simulink model "S_GITHUB"  (R2017a)
settings: Solver=VariableStepAuto  StartTime=0.0  StopTime=20  FixedStep=1e-6  MaxStep=1e-4
values from neighbouring files (symbols this model uses):
  Cinv = 470e-6    (= 0.00047)    [M_GITHUB.m]
  Co = 470e-6    (= 0.00047)    [M_GITHUB.m]
  Den = 1.225    [M_GITHUB.m]
  Dg = 0.390    (= 0.39)    [M_GITHUB.m]
  Dmax = 1    [M_GITHUB.m]
  Jg = 5*0.1    (= 0.5)    [M_GITHUB.m]
  Jm = 5*0.1    (= 0.5)    [M_GITHUB.m]
  KI = 0.0195296    [M_GITHUB.m]
  Ki1 = 1/io_nom    (= 0.0444444444444)    [M_GITHUB.m]
  KP = 1.0672352    [M_GITHUB.m]
  L = 80e-3    (= 0.08)    [M_GITHUB.m]
  Rr = 2.9343    [M_GITHUB.m]
  Rs1 = 2.5    [M_GITHUB.m]
  Ts1 = 1/Fs1    (= 0.0002)    [M_GITHUB.m]
undefined symbols (not defined in the file or in its folder): Ion, Lithium, RL
undefined symbols (not defined in the file): Fs1
libraries: powerlib x18, fuzblock x3, simulink x2, electricdrivelib x1, simulink_extras x1
settings Model: ExtModeTrigDuration=10  Creator=dricl  LastModifiedBy=dricl
settings SolverCC: MaxConsecutiveZCs=10000000
settings OptimizationCC: PassReuseOutputArgsAs=Individual arguments  MaxStackSize=2560
settings DebuggingCC: ParameterTunabilityLossMsg=error
settings HardwareCC: ProdBitPerPointer=32  ProdBitPerSizeT=32  ProdBitPerPtrDiffT=32  ProdLargestAtomicInteger=Long  ProdLargestAtomicFloat=Double  ProdWordSize=32  ProdLongLongMode=on  ProdHWDeviceType=ARM Compatible->ARM Cortex
settings SFSimCC: MATLABDynamicMemAlloc=off
settings RTWCC: SystemTargetFile=ert.tlc  HardwareBoard=TI Concerto F28M35x (ARM Cortex-M3)  TLCOptions=-aInlineSetEventsForThisBaseRateFcn=TLC_FALSE -aSuppressMultiTaskScheduler=TLC_FALSE -aRateBasedStepFcn=1  TemplateMakefile=ert_default_tmf  Description=Embedded Coder  GenerateReport=on  Toolchain=Texas Instruments Code Composer Studio v6 (ARM)  IncludeHyperlinkInReport=on  LaunchReport=on  CreateSILPILBlock=PIL  GenerateTraceInfo=on  GenerateTraceReport=on  GenerateTraceReportSl=on  GenerateTraceReportSf=on  GenerateTraceReportEml=on
settings CodeAppCC: ForceParamTrailComments=on  IgnoreCustomStorageClasses=off  OperatorAnnotations=on  SimulinkDataObjDesc=on  SFDataObjDesc=on  MATLABFcnDesc=on  InsertBlockDesc=on  MATLABSourceComments=on

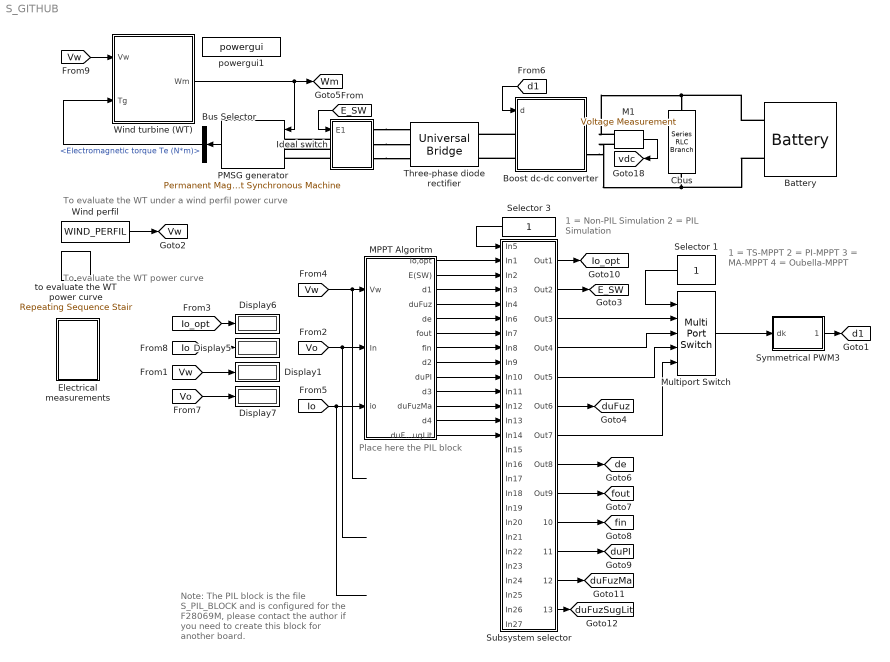
== system S_GITHUB ==
  note: Place here the
      | PIL block
  note: 1 = TS-MPPT
      | 2 = PI-MPPT
      | 3 = MA-MPPT
      | 4 = Oubella-MPPT
  note: 1 = Non-PIL Simulation
      | 2 = PIL Simulation
  note: Note: The PIL block is the file S_PIL_BLOCK and is configured for the F28069M, please contact the author if you need to create this block for another board.
  note: To evaluate the WT under a wind perfil power curve
  note: To evaluate the WT power curve
  Battery : electricdrivelib/Extra Sources/Battery  BatType=Lithium-Ion  ShowTempParam=off  ThermalPreset=no  ShowAgeParam=off  NomV=500  NomQ=5.4  SOC=20  Batt_Tr=30  PresetModel=on  MaxQ=5.4  MinV=375  FullV=581.9936  Dis_rate=2.3478  R=0.92593  Normal_OP=4.8835  expZone="[540.1929     0.2653043]"  current=[6.5 13 32.5]  Units=Time  Tci=20  NomT=20  T2=-30  MaxQ2=4.8  FullV2=7.1  Normal_OP2=5.655  expZone2="[6.58           1]"  Rca=0.6  ti=2000  Dp=0  Neq0=0  Tsim=1e6  Ta1=25  Qeol=5.4*0.9  Reol=0.013333*1.2  Char_age=[2.3478, 3]  Dis_age=[2.3478, 10]  N1=1500  N2=10500  N3=1000  N4=1400  Ta2=45  N5=950
  Boost dc-dc converter : Subsystem
  Bus Selector : BusSelector  OutputSignals=Electromagnetic torque Te (N*m)
  Cbus : powerlib/Elements/Series RLC Branch  LConnTagsString=__new0  RConnTagsString=__new0  BranchType=RC  Resistance=0.01  Inductance=1e-3  SetiL0=off  InitialCurrent=0  Capacitance=Cinv  Setx0=on  InitialVoltage=0  Measurements=None
  Display{1,5..7} (4 alike) : Display
  Electrical measurements : Subsystem
  Ideal switch : Subsystem
  M1 : powerlib/Measurements/Voltage Measurement  PhasorSimulation=off  OutputType=Complex  PSBequivalent=0
  MPPT Algoritm : Subsystem
  Multiport Switch : MultiPortSwitch  Inputs=4
  PMSG generator : powerlib/Machines/Permanent Magnet Synchronous Machine  NbPhases=3  FluxDistribution=Sinusoidal  RotorType=Round  MechanicalLoad=Speed w  PresetModel=No  ShowDetailedParameters=on  MeasurementBus=off  Resistance=Rs1  Inductance=8.5e-3  dqInductances=[0.0007552 0.0008348]  La=La  MachineConstant=Flux linkage established by magnets (V.s)  Flux=Ym  VoltageCst=2176.5592  TorqueCst=18  Flat=120  Mechanical=[0.011 0.001417 4 0]  PolePairs=p  InitialConditions=[0,0, 0,0]  InitialConditions5ph=[0 0 0 0 0 0]  TsPowergui=0  TsBlock=-1  RefAngle=90 degrees behind phase A axis (modified Park)
      settings: SourceProductName=Simscape Power Systems
  Selector 1 : Constant
  Selector 3 : Constant
  Subsystem selector : Subsystem
  Symmetrical PWM3 : Subsystem  AncestorBlock=plecslib_extras2/Modulators/Symmetrical PWM  mask(Symmetrical PWM){sampling=Natural (carrier starts with 0), fc=Fs1, offset=0, input_limits=[0 Dmax], output_values=[0 1]}
      mask prompts: fc "Carrier frequency (Hz):"; offset "Carrier offset (p.u.):"; input_limits "Input limits [min max]:"; output_values "Output values [off on]:"
      mask help: PWM generator with a symmetrical triangular carrier. If the input is a vector, the output is also a vector of the same width.
      mask init:
      | if numel(fc)>1 || fc<=0,
      |   error('Carrier frequency must be a positive scalar.');
      | end
      | if numel(offset)>1 || offset<0 || offset>=1,
      |   error('Carrier offset must be a scalar in the range [0; 1/fc[.');
      | end
      | if sampling == 1,
      |   offset = mod(offset+.75, 1);
      | end
      | 
      | si = [.5 mod(offset, .5)]/fc;
      mask Help: eval('plecs(''help'', ''symmetricalpwm.html'')')
      mask TypeOptions sampling: Natural (carrier starts with 0) | Natural (carrier starts with 1) | Regular (double edge) | Regular (single edge)
  Three-phase diode rectifier : powerlib/Power Electronics/Universal Bridge  Arms=3  SnubberResistance=Rs2  SnubberCapacitance=Cs  Device=Diodes  Ron=Ron  Lon=0  ForwardVoltages="[  0  0  ]"  ForwardVoltage=0.7  GTOparameters=[ 10e-6 , 20e-6 ]  IGBTparameters=[ 1e-6 , 2e-6 ]  Measurements=None  Measurements_2=None  converterType=Rectifier
  Wind perfil : FromWorkspace  VariableName=WIND_PERFIL
  Wind turbine (WT) : Subsystem
      mask Display: image('Rotor.jpg');
  powergui1 : powerlib/powergui  Priority=1  SimulationMode=Continuous  SampleTime=1e-6  frequency=60  Iterations=50  frequencyindice=0  Pbase=100e6  ErrMax=1e-4  UnitsV=kV  UnitsW=MW  buscounter=0  FunctionMessages=off  echomessages=off  EnableUseOfTLC=off  CurrentSourceSwitches=off  DisableSnubberDevices=off  DisableRonSwitches=off  DisableVfSwitches=off  DisplayEquations=off  SolverType=Tustin/Backward Euler (TBE)  Interpol=off  ExternalGateDelay=off  methode=off  Ts=100  x0status=blocks  SPID=on  SwTol=0  HookPort=off  RestoreLinks=warning  ResistiveCurrentMeasurement=off  Frange=[0:2:500]  Ylog=off  Xlog=on  ShowGrid=off  save=off  variable=ZData  structure=0  ZoomFFT=off  StartTime=0.0  cycles=1  DisplayStyle=1  fundamental=60  FreqAxis=off  MaxFrequency=1000  frequencyindicesteady=1  RmsSteady=1  display=off
  to evaluate the WT power curve : simulink/Sources/Repeating Sequence Stair  OutValues=[12 12 14 16 16.8 18 18 14 14 2 2 14 14].'  tsamp=1  OutMin=[]  OutMax=[]  OutDataTypeStr=double  OutputDataTypeScalingMode=double  OutDataType=fixdt(0,8)  ConRadixGroup=Best Precision: Vector-wise  OutScaling=2^-12
  tag scope: E_SW=global, Io_opt=global, Vw=global, Wm=global, d1=global, de=global, duFuz=global, duFuzMa=global, duFuzSugLit=global, duPI=global, fin=global, fout=global, vdc=global
  wires:
  Wind turbine (WT)/1(Wm) -> [Wm], PMSG generator/1
  Bus Selector/1 -> Wind turbine (WT)/2(Tg)  "<Electromagnetic torque Te (N*m)>"
  PMSG generator/1 -> Bus Selector/1
  M1/1 -> [vdc]
  [d1] -> Boost dc-dc converter/1(d)
  [Vw] -> Wind turbine (WT)/1(Vw)
  [Vo] -> Display7/1
  [Vw] -> Display1/1
  [E_SW] -> Ideal switch/1(E1)
  [Io_opt] -> Display6/1
  [Io] -> Display5/1
  [Vw] -> MPPT Algoritm/1(Vw)
  [Io] -> MPPT Algoritm/3(io)
  [Vo] -> MPPT Algoritm/2(In)
  Symmetrical PWM3/1(dmppt) -> [d1]
  Multiport Switch/1 -> Symmetrical PWM3/1(dk)
  Selector 1/1 -> Multiport Switch/1
  MPPT Algoritm/1(Io,opt) -> Subsystem selector/2(In1)
  MPPT Algoritm/2(E(SW)) -> Subsystem selector/3(In2)
  MPPT Algoritm/3(d1) -> Subsystem selector/4(In3)
  MPPT Algoritm/4(duFuz) -> Subsystem selector/5(In4)
  Selector 3/1 -> Subsystem selector/1(In5)
  MPPT Algoritm/5(de) -> Subsystem selector/6(In6)
  MPPT Algoritm/6(fout) -> Subsystem selector/7(In7)
  MPPT Algoritm/7(fin) -> Subsystem selector/8(In8)
  MPPT Algoritm/8(d2) -> Subsystem selector/9(In9)
  MPPT Algoritm/9(duPI) -> Subsystem selector/10(In10)
  MPPT Algoritm/10(d3) -> Subsystem selector/11(In11)
  MPPT Algoritm/11(duFuzMa) -> Subsystem selector/12(In12)
  MPPT Algoritm/12(d4) -> Subsystem selector/13(In13)
  MPPT Algoritm/13(duFuzSugLit) -> Subsystem selector/14(In14)
  ? -> Subsystem selector/15(In15)
  ? -> Subsystem selector/16(In16)
  ? -> Subsystem selector/17(In17)
  ? -> Subsystem selector/18(In18)
  ? -> Subsystem selector/19(In19)
  ? -> Subsystem selector/20(In20)
  ? -> Subsystem selector/21(In21)
  ? -> Subsystem selector/22(In22)
  ? -> Subsystem selector/23(In23)
  ? -> Subsystem selector/24(In24)
  ? -> Subsystem selector/25(In25)
  ? -> Subsystem selector/27(In27)
  Subsystem selector/1(Out1) -> [Io_opt]
  Subsystem selector/2(Out2) -> [E_SW]
  Subsystem selector/3(Out3) -> Multiport Switch/2
  Subsystem selector/4(Out4) -> Multiport Switch/3
  Subsystem selector/5(Out5) -> Multiport Switch/4
  Subsystem selector/6(Out6) -> [duFuz]
  Subsystem selector/7(Out7) -> Multiport Switch/5
  Subsystem selector/8(Out8) -> [de]
  Subsystem selector/9(Out9) -> [fout]
  Subsystem selector/10(Out10) -> [fin]
  Subsystem selector/11(Out11) -> [duPI]
  Subsystem selector/12(Out12) -> [duFuzMa]
  Subsystem selector/13(Out13) -> [duFuzSugLit]
  ? -> Subsystem selector/26(In26)
  Wind perfil/1 -> [Vw]
  connections:
  M1/LConn1 -- Boost dc-dc converter/RConn1 -- Battery/LConn1 -- Cbus/LConn1
  M1/LConn2 -- Boost dc-dc converter/RConn2 -- Battery/LConn2 -- Cbus/RConn1
  Boost dc-dc converter/LConn1 -- Three-phase diode rectifier/RConn1
  Boost dc-dc converter/LConn2 -- Three-phase diode rectifier/RConn2
  Ideal switch/LConn2 -- PMSG generator/LConn2
  Ideal switch/LConn3 -- PMSG generator/LConn3
  Ideal switch/LConn1 -- PMSG generator/LConn1
  Ideal switch/RConn1 -- Three-phase diode rectifier/LConn1
  Ideal switch/RConn2 -- Three-phase diode rectifier/LConn2
  Ideal switch/RConn3 -- Three-phase diode rectifier/LConn3

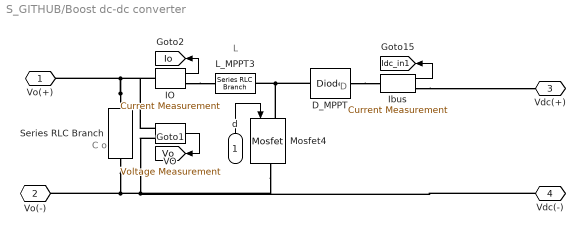
== system S_GITHUB/Boost dc-dc converter ==
  note: C o
  note: L
  note: D
  d : Inport
  D_MPPT : powerlib/Power Electronics/Diode  Ron=0.001  Lon=0  Vf=0.7  IC=0  UseSnubber=0  Rs=1e5  Cs=inf  Measurements=off
  IO : powerlib/Measurements/Current Measurement  PhasorSimulation=off  OutputType=Complex  PSBequivalent=0
  Ibus : powerlib/Measurements/Current Measurement  PhasorSimulation=off  OutputType=Complex  PSBequivalent=0
  L_MPPT3 : powerlib/Elements/Series RLC Branch  LConnTagsString=__new0  RConnTagsString=__new0  BranchType=L  Resistance=RL  Inductance=L  SetiL0=off  InitialCurrent=0  Capacitance=1e-6  Setx0=off  InitialVoltage=0  Measurements=None
  Mosfet4 : powerlib/Power Electronics/Mosfet  Ron=0.001  Lon=0  Rd=0.001  Vfd=0.7  IC=0  Rs=1e5  Cs=inf  Measurements=off
  Series RLC Branch : powerlib/Elements/Series RLC Branch  LConnTagsString=__new0  RConnTagsString=__new0  BranchType=RC  Resistance=0.01  Inductance=1e-3  SetiL0=off  InitialCurrent=0  Capacitance=Co  Setx0=on  InitialVoltage=0  Measurements=None
  VO : powerlib/Measurements/Voltage Measurement  PhasorSimulation=off  OutputType=Complex  PSBequivalent=0
  Vo(+) : PMIOPort  Port=1  Side=Left
  Vo(-) : PMIOPort  Port=2  Side=Left
  Vdc(+) : PMIOPort  Port=3  Side=Right
  Vdc(-) : PMIOPort  Port=4  Side=Right
  tag scope: Idc_in1=global, Io=global, Vo=global
  wires:
  IO/1 -> [Io]
  VO/1 -> [Vo]
  d/1 -> Mosfet4/1
  Ibus/1 -> [Idc_in1]
  connections:
  Ibus/RConn1 -- Vdc(+)/RConn1
  Series RLC Branch/LConn1 -- Vo(+)/RConn1 -- IO/LConn1 -- VO/LConn1
  Series RLC Branch/RConn1 -- Vdc(-)/RConn1 -- Mosfet4/RConn1 -- VO/LConn2 -- Vo(-)/RConn1
  IO/RConn1 -- L_MPPT3/LConn1
  D_MPPT/RConn1 -- Ibus/LConn1
  Mosfet4/LConn1 -- D_MPPT/LConn1 -- L_MPPT3/RConn1

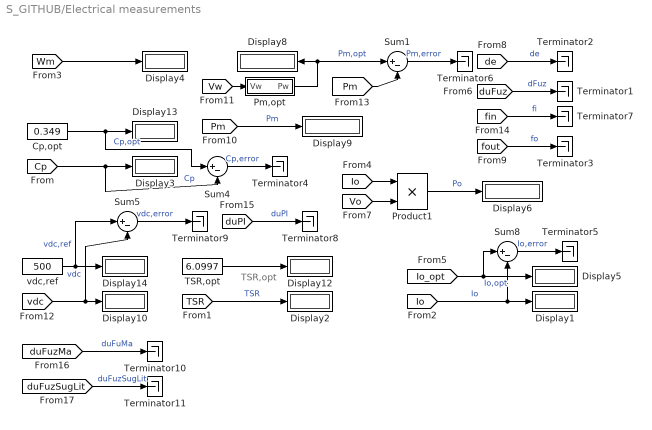
== system S_GITHUB/Electrical measurements ==
  note: TSR,opt
  Cp,opt : Constant  Value=0.349
  Display{1..6,8..10,12..14} (12 alike) : Display
  Pm,opt : MATLAB Function  TreatAsAtomicUnit=on
  Product1 : Product
  Sum{1,4..5,8} (4 alike) : Sum  Inputs=|+-
  TSR,opt : Constant  Value=6.0997
  Terminator{1..11} (11 alike) : Terminator
  vdc,ref : Constant  Value=500
  wires:
  Sum5/1 -> Terminator9/1  "vdc,error"
  vdc,ref/1 -> Sum5/1, Display14/1  "vdc,ref"
  TSR,opt/1 -> Display12/1
  Cp,opt/1 -> Sum4/1, Display13/1  "Cp,opt"
  Sum4/1 -> Terminator4/1  "Cp,error"
  [Pm] -> Sum1/2
  Sum1/1 -> Terminator6/1  "Pm,error"
  [Wm] -> Display4/1
  [TSR] -> Display2/1  "TSR"
  [Cp] -> Sum4/2, Display3/1  "Cp"
  Pm,opt/1(Pw) -> Display8/1, Sum1/1  "Pm,opt"
  [Vw] -> Pm,opt/1(Vw)
  [Pm] -> Display9/1  "Pm"
  [vdc] -> Sum5/2, Display10/1  "vdc"
  [Io_opt] -> Sum8/1, Display5/1  "Io,opt"
  Sum8/1 -> Terminator5/1  "Io,error"
  [Io] -> Sum8/2, Display1/1  "Io"
  [Io] -> Product1/1
  [Vo] -> Product1/2
  Product1/1 -> Display6/1  "Po"
  [duFuz] -> Terminator1/1  "dFuz"
  [de] -> Terminator2/1  "de"
  [fout] -> Terminator3/1  "fo"
  [fin] -> Terminator7/1  "fi"
  [duPI] -> Terminator8/1  "duPI"
  [duFuzMa] -> Terminator10/1  "duFuMa"
  [duFuzSugLit] -> Terminator11/1  "duFuzSugLit"

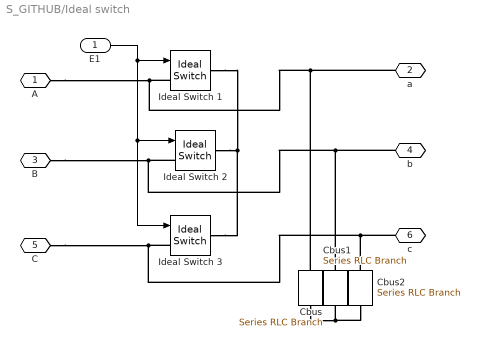
== system S_GITHUB/Ideal switch ==
  E1 : Inport
  Cbus : powerlib/Elements/Series RLC Branch  LConnTagsString=__new0  RConnTagsString=__new0  BranchType=R  Resistance=100000  Inductance=1e-3  SetiL0=off  InitialCurrent=0  Capacitance=Cinv  Setx0=on  InitialVoltage=0  Measurements=None
  Cbus1 : powerlib/Elements/Series RLC Branch  LConnTagsString=__new0  RConnTagsString=__new0  BranchType=R  Resistance=100000  Inductance=1e-3  SetiL0=off  InitialCurrent=0  Capacitance=Cinv  Setx0=on  InitialVoltage=0  Measurements=None
  Cbus2 : powerlib/Elements/Series RLC Branch  LConnTagsString=__new0  RConnTagsString=__new0  BranchType=R  Resistance=100000  Inductance=1e-3  SetiL0=off  InitialCurrent=0  Capacitance=Cinv  Setx0=on  InitialVoltage=0  Measurements=None
  Ideal Switch 1 : powerlib/Power Electronics/Ideal Switch  Ron=0.001  Lon=1e-9  IC=1  Rs=1e6  Cs=100e-9  Measurements=off
      settings: AttributesFormatString=\n
  Ideal Switch 2 : powerlib/Power Electronics/Ideal Switch  Ron=0.001  Lon=1e-9  IC=1  Rs=inf  Cs=0  Measurements=off
      settings: AttributesFormatString=\n
  Ideal Switch 3 : powerlib/Power Electronics/Ideal Switch  Ron=0.001  Lon=1e-9  IC=1  Rs=inf  Cs=0  Measurements=off
      settings: AttributesFormatString=\n
  A : PMIOPort  Port=1  Side=Left
  a : PMIOPort  Port=2  Side=Right
  B : PMIOPort  Port=3  Side=Left
  b : PMIOPort  Port=4  Side=Right
  C : PMIOPort  Port=5  Side=Left
  c : PMIOPort  Port=6  Side=Right
  wires:
  E1/1 -> Ideal Switch 3/1, Ideal Switch 2/1, Ideal Switch 1/1
  connections:
  C/RConn1 -- Ideal Switch 3/LConn1 -- Cbus2/LConn1 -- c/RConn1
  B/RConn1 -- Ideal Switch 2/LConn1 -- Cbus1/LConn1 -- b/RConn1
  A/RConn1 -- Cbus/LConn1 -- a/RConn1 -- Ideal Switch 1/LConn1
  Ideal Switch 1/RConn1 -- Ideal Switch 3/RConn1 -- Ideal Switch 2/RConn1
  Cbus2/RConn1 -- Cbus/RConn1 -- Cbus1/RConn1

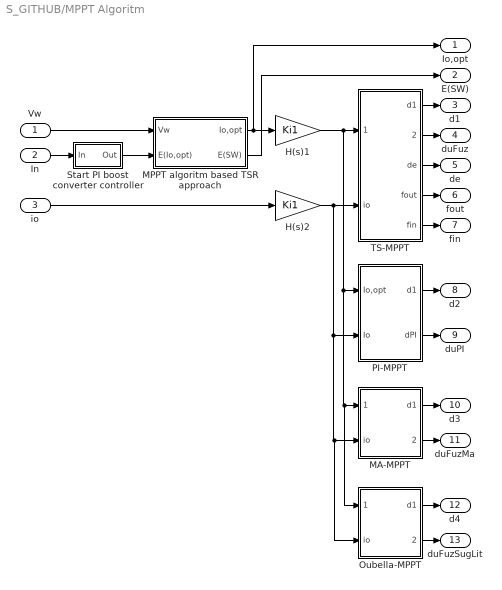
== system S_GITHUB/MPPT Algoritm ==
  Vw : Inport
  In : Inport  Port=2
  io : Inport  Port=3
  H(s)1 : Gain  Gain=Ki1
  H(s)2 : Gain  Gain=Ki1
  MA-MPPT : Subsystem
  "MPPT algoritm based TSR approach " : Subsystem
  Oubella-MPPT : Subsystem
  PI-MPPT : Subsystem
  Start PI boost converter controller : Subsystem
  TS-MPPT : Subsystem
  Io,opt : Outport
  E(SW) : Outport  Port=2
  d1 : Outport  Port=3
  duFuz : Outport  Port=4
  de : Outport  Port=5
  fout : Outport  Port=6
  fin : Outport  Port=7
  d2 : Outport  Port=8
  duPI : Outport  Port=9
  d3 : Outport  Port=10
  duFuzMa : Outport  Port=11
  d4 : Outport  Port=12
  duFuzSugLit : Outport  Port=13
  wires:
  H(s)2/1 -> Oubella-MPPT/2(io), MA-MPPT/2(io), PI-MPPT/2(Io), TS-MPPT/2(io)
  H(s)1/1 -> Oubella-MPPT/1(io,opt), MA-MPPT/1(io,opt), PI-MPPT/1(Io,opt), TS-MPPT/1(io,opt)
  "MPPT algoritm based TSR approach "/1(Io,opt) -> Io,opt/1, H(s)1/1
  io/1 -> H(s)2/1
  "MPPT algoritm based TSR approach "/2(E(SW)) -> E(SW)/1
  Start PI boost converter controller/1(Out) -> "MPPT algoritm based TSR approach "/2(E(Io,opt))
  TS-MPPT/5(fin) -> fin/1
  TS-MPPT/3(de) -> de/1
  TS-MPPT/2(duFuz) -> duFuz/1
  TS-MPPT/4(fout) -> fout/1
  In/1 -> Start PI boost converter controller/1(In)
  Vw/1 -> "MPPT algoritm based TSR approach "/1(Vw)
  TS-MPPT/1(d1) -> d1/1
  PI-MPPT/1(d1) -> d2/1
  PI-MPPT/2(dPI) -> duPI/1
  MA-MPPT/1(d1) -> d3/1
  MA-MPPT/2(duFuzMa) -> duFuzMa/1
  Oubella-MPPT/1(d1) -> d4/1
  Oubella-MPPT/2(duFuzMa) -> duFuzSugLit/1

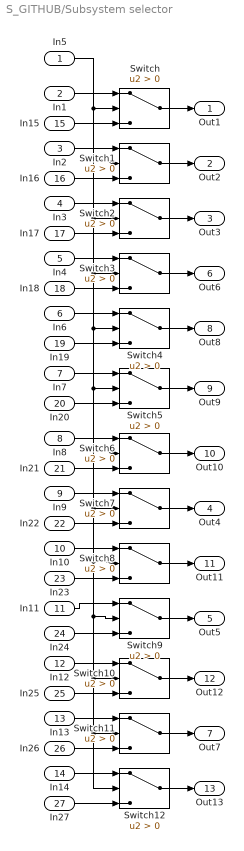
== system S_GITHUB/Subsystem selector ==
  In5 : Inport
  In1 : Inport  Port=2
  In2 : Inport  Port=3
  In3 : Inport  Port=4
  In4 : Inport  Port=5
  In6 : Inport  Port=6
  In7 : Inport  Port=7
  In8 : Inport  Port=8
  In9 : Inport  Port=9
  In10 : Inport  Port=10
  In11 : Inport  Port=11
  In12 : Inport  Port=12
  In13 : Inport  Port=13
  In14 : Inport  Port=14
  In15 : Inport  Port=15
  In16 : Inport  Port=16
  In17 : Inport  Port=17
  In18 : Inport  Port=18
  In19 : Inport  Port=19
  In20 : Inport  Port=20
  In21 : Inport  Port=21
  In22 : Inport  Port=22
  In23 : Inport  Port=23
  In24 : Inport  Port=24
  In25 : Inport  Port=25
  In26 : Inport  Port=26
  In27 : Inport  Port=27
  Switch{,1..12} (13 alike) : Switch  Criteria=u2 > Threshold
  Out1 : Outport
  Out2 : Outport  Port=2
  Out3 : Outport  Port=3
  Out4 : Outport  Port=4
  Out5 : Outport  Port=5
  Out6 : Outport  Port=6
  Out7 : Outport  Port=7
  Out8 : Outport  Port=8
  Out9 : Outport  Port=9
  Out10 : Outport  Port=10
  Out11 : Outport  Port=11
  Out12 : Outport  Port=12
  Out13 : Outport  Port=13
  wires:
  Switch12/1 -> Out13/1
  In26/1 -> Switch11/3
  In13/1 -> Switch11/1
  Switch11/1 -> Out7/1
  In14/1 -> Switch12/1
  Switch9/1 -> Out5/1
  Switch2/1 -> Out3/1
  Switch7/1 -> Out4/1
  In21/1 -> Switch6/3
  In23/1 -> Switch8/3
  Switch/1 -> Out1/1
  Switch4/1 -> Out8/1
  Switch1/1 -> Out2/1
  In11/1 -> Switch9/1
  Switch6/1 -> Out10/1
  Switch8/1 -> Out11/1
  Switch5/1 -> Out9/1
  Switch3/1 -> Out6/1
  In20/1 -> Switch5/3
  In25/1 -> Switch10/3
  In5/1 -> Switch/2, Switch1/2, Switch2/2, Switch3/2, Switch4/2, Switch5/2, Switch6/2, Switch7/2, Switch8/2, Switch9/2, Switch10/2, Switch11/2, Switch12/2
  In27/1 -> Switch12/3
  In16/1 -> Switch1/3
  In12/1 -> Switch10/1
  Switch10/1 -> Out12/1
  In24/1 -> Switch9/3
  In15/1 -> Switch/3
  In6/1 -> Switch4/1
  In9/1 -> Switch7/1
  In10/1 -> Switch8/1
  In17/1 -> Switch2/3
  In8/1 -> Switch6/1
  In18/1 -> Switch3/3
  In3/1 -> Switch2/1
  In2/1 -> Switch1/1
  In4/1 -> Switch3/1
  In7/1 -> Switch5/1
  In1/1 -> Switch/1
  In19/1 -> Switch4/3
  In22/1 -> Switch7/3

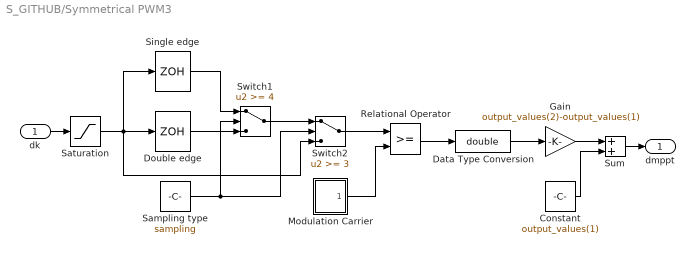
== system S_GITHUB/Symmetrical PWM3 ==
  dk : Inport
  Constant : Constant  Value=output_values(1)
  Data Type Conversion : DataTypeConversion  OutDataTypeStr=double  SaturateOnIntegerOverflow=on  RndMeth=Zero
  Double edge : ZeroOrderHold  SampleTime=si
  Gain : Gain  Gain=output_values(2)-output_values(1)  SaturateOnIntegerOverflow=on  OutDataTypeStr=Inherit: Same as input  ParamDataTypeStr=Inherit: Same as input
  Modulation Carrier : Subsystem  mask(Symmetric Triangle Generator){fc=fc, offset=mod(offset+.5, 1), range=input_limits}
      mask prompts: fc "Carrier frequency (Hz):"; offset "Carrier offset (p.u.):"; range "Signal range [min max]:"
      mask help: Generates a symmetrical triangular signal with output values between 0 and 1. The block forces the Simulink solver to output all tips of the signal. The output can therefore be used as a carrier signal for PWM.
      mask init:
      | if numel(fc)>1 || fc<=0,
      |   error('Carrier frequency must be a positive scalar.');
      | end
      | if numel(offset)>1 || offset<0 || offset>=1,
      |   error('Carrier offset must be a scalar in the interval [0; 1[.');
      | end
      | if numel(range)~=2,
      |   error('Signal range must be a two-element vector.')
      | end
      | if range(1)>=range(2),
      |   error('Signal range must be specified as [min max].')
      | end
      | 
      | carrier_t = [0 offset mod(1/2+offset, 1) 1]/fc;
      | carrier_v0 = 1-2*abs(offset-.5);
      | carrier_v = range(1)+[carrier_v0 0 1 carrier_v0]*diff(range);
      | [carrier_t, idx] = unique(carrier_t);
      | carrier_v = carrier_v(idx);
      | si = [.5 mod(offset, .5)]/fc;
      | 
      | L = length(carrier_t);
      | disp_seq_t = repmat(carrier_t(:),1,3) + ones(L,1)*[0,1,2]/fc;
      | disp_seq_v = repmat(carrier_v(:),1,3);
      mask Display: plot(disp_seq_t, disp_seq_v)
  Relational Operator : RelationalOperator  RndMeth=Nearest  InputSameDT=on
  Sampling type : Constant  Value=sampling
  Saturation : Saturate  UpperLimit=input_limits(2)  LowerLimit=input_limits(1)
  Single edge : ZeroOrderHold  SampleTime=[1 offset]/fc
  Sum : Sum  SaturateOnIntegerOverflow=on  InputSameDT=on  OutDataTypeStr=Inherit: Same as first input
  Switch1 : Switch  Threshold=4  SaturateOnIntegerOverflow=on  InputSameDT=on
  Switch2 : Switch  Threshold=3  SaturateOnIntegerOverflow=on  InputSameDT=on
  dmppt : Outport
  wires:
  Data Type Conversion/1 -> Gain/1
  Constant/1 -> Sum/2
  Gain/1 -> Sum/1
  Sum/1 -> dmppt/1
  Relational Operator/1 -> Data Type Conversion/1
  Switch2/1 -> Relational Operator/1
  Sampling type/1 -> Switch1/2, Switch2/2
  Single edge/1 -> Switch1/1
  Saturation/1 -> Double edge/1, Single edge/1, Switch2/3
  dk/1 -> Saturation/1
  Modulation Carrier/1(Out) -> Relational Operator/2
  Switch1/1 -> Switch2/1
  Double edge/1 -> Switch1/3

== system S_GITHUB/Wind turbine (WT) ==
  Vw : Inport
  Tg : Inport  Port=2
  Theoretical maximum power : MATLAB Function  TreatAsAtomicUnit=on
  WT dynamic model : Subsystem
  WT static model : Subsystem
  Wm : Outport
  tag scope: Cp=global, Pm=global, Pw=global, TSR=global, Tm=global
  wires:
  WT static model/1(Pm) -> [Pm]
  WT static model/3(Cp) -> [Cp]
  WT static model/4(Tm) -> WT dynamic model/1(Tm), [Tm]
  Tg/1 -> WT dynamic model/2(Tg)
  Theoretical maximum power/1(Pw) -> [Pw]
  WT static model/2(TSR) -> [TSR]
  Vw/1 -> Theoretical maximum power/1(Vw), WT static model/1(Vw)
  WT dynamic model/1(Wm) -> WT static model/2(Wm), Wm/1

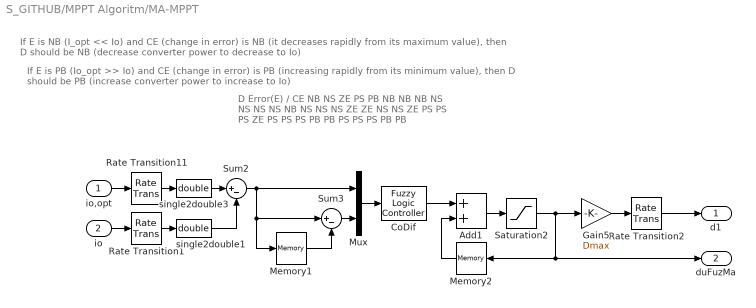
== system S_GITHUB/MPPT Algoritm/MA-MPPT ==
  note: If E is PB (Io_opt >> Io) and CE (change in error) is PB (increasing rapidly from its minimum value), then D should be PB (increase converter power to increase to Io)
  note: If E is NB (I_opt << Io) and CE (change in error) is NB (it decreases rapidly from its maximum value), then D should be NB (decrease converter power to decrease to Io)
  note: D
      | Error(E) / CE NB NS ZE PS PB
      | NB NB NB NS NS NS
      | NS NB NS NS NS ZE
      | ZE NS NS ZE PS PS
      | PS ZE PS PS PS PB
      | PB PS PS PS PB PB
  io,opt : Inport
  io : Inport  Port=2
  Add1 : Sum
  CoDif : fuzblock/Fuzzy Logic  Controller  fis=['MA_MPPT.fis']
  Gain5 : Gain  Gain=Dmax
  Memory1 : Memory  InheritSampleTime=on
  Memory2 : Memory  InheritSampleTime=on
  Mux : Mux  Inputs=2
  Rate Transition1 : RateTransition  Deterministic=off  OutPortSampleTime=Ts6
  Rate Transition11 : RateTransition  Deterministic=off  OutPortSampleTime=Ts6
  Rate Transition2 : RateTransition  Deterministic=off  OutPortSampleTime=Ts6
  Saturation2 : Saturate  UpperLimit=0.98  LowerLimit=0.01
  Sum2 : Sum  Inputs=|+-
  Sum3 : Sum  Inputs=|+-
  single2double1 : DataTypeConversion  OutDataTypeStr=double
  single2double3 : DataTypeConversion  OutDataTypeStr=double
  d1 : Outport
  duFuzMa : Outport  Port=2
  wires:
  Rate Transition2/1 -> d1/1
  Rate Transition11/1 -> single2double3/1
  Sum2/1 -> Sum3/1, Memory1/1, Mux/1
  Memory2/1 -> Add1/2
  single2double3/1 -> Sum2/1
  Mux/1 -> CoDif/1
  Sum3/1 -> Mux/2
  single2double1/1 -> Sum2/2
  Memory1/1 -> Sum3/2
  Rate Transition1/1 -> single2double1/1
  io,opt/1 -> Rate Transition11/1
  io/1 -> Rate Transition1/1
  Gain5/1 -> Rate Transition2/1
  Add1/1 -> Saturation2/1
  Saturation2/1 -> Gain5/1, duFuzMa/1, Memory2/1
  CoDif/1 -> Add1/1

== system S_GITHUB/MPPT Algoritm/MPPT algoritm based TSR approach  ==
  Vw : Inport
  E(Io,opt) : Inport  Port=2
  "Io,opt estimator " : MATLAB Function  TreatAsAtomicUnit=on
  Product : Product
  Rate Transition1 : RateTransition  Deterministic=off  OutPortSampleTime=Ts1
  Rate Transition11 : RateTransition  Deterministic=off  OutPortSampleTime=Ts1
  Wm,opt computation : MATLAB Function  TreatAsAtomicUnit=on
  single2double1 : DataTypeConversion  OutDataTypeStr=double
  Io,opt : Outport
  E(SW) : Outport  Port=2
  wires:
  Wm,opt computation/1(y) -> "Io,opt estimator "/1(y)
  Vw/1 -> Rate Transition11/1
  Rate Transition11/1 -> single2double1/1
  single2double1/1 -> Wm,opt computation/1(x)
  "Io,opt estimator "/2(E) -> E(SW)/1
  "Io,opt estimator "/1(x) -> Product/2
  Product/1 -> Io,opt/1
  E(Io,opt)/1 -> Rate Transition1/1
  Rate Transition1/1 -> Product/1

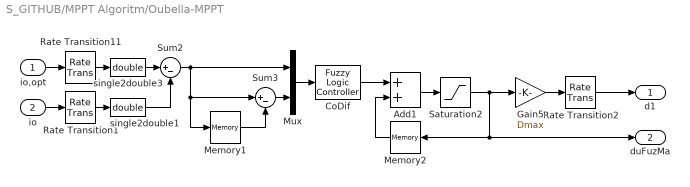
== system S_GITHUB/MPPT Algoritm/Oubella-MPPT ==
  io,opt : Inport
  io : Inport  Port=2
  Add1 : Sum
  CoDif : fuzblock/Fuzzy Logic  Controller  fis=['OUBELLA_MPPT.fis']
  Gain5 : Gain  Gain=Dmax
  Memory1 : Memory  InheritSampleTime=on
  Memory2 : Memory  InheritSampleTime=on
  Mux : Mux  Inputs=2
  Rate Transition1 : RateTransition  Deterministic=off  OutPortSampleTime=Ts6
  Rate Transition11 : RateTransition  Deterministic=off  OutPortSampleTime=Ts6
  Rate Transition2 : RateTransition  Deterministic=off  OutPortSampleTime=Ts6
  Saturation2 : Saturate  UpperLimit=0.98  LowerLimit=0.01
  Sum2 : Sum  Inputs=|+-
  Sum3 : Sum  Inputs=|+-
  single2double1 : DataTypeConversion  OutDataTypeStr=double
  single2double3 : DataTypeConversion  OutDataTypeStr=double
  d1 : Outport
  duFuzMa : Outport  Port=2
  wires:
  Rate Transition2/1 -> d1/1
  Rate Transition11/1 -> single2double3/1
  Sum2/1 -> Sum3/1, Memory1/1, Mux/1
  Memory2/1 -> Add1/2
  single2double3/1 -> Sum2/1
  Mux/1 -> CoDif/1
  Sum3/1 -> Mux/2
  single2double1/1 -> Sum2/2
  Memory1/1 -> Sum3/2
  Rate Transition1/1 -> single2double1/1
  io,opt/1 -> Rate Transition11/1
  io/1 -> Rate Transition1/1
  Gain5/1 -> Rate Transition2/1
  Add1/1 -> Saturation2/1
  Saturation2/1 -> Gain5/1, duFuzMa/1, Memory2/1
  CoDif/1 -> Add1/1

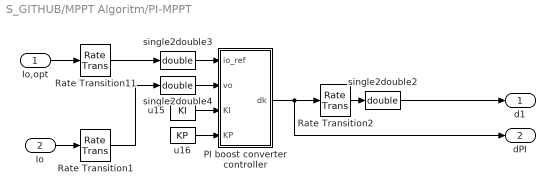
== system S_GITHUB/MPPT Algoritm/PI-MPPT ==
  Io,opt : Inport
  Io : Inport  Port=2
  PI boost converter controller : MATLAB Function  TreatAsAtomicUnit=on
  Rate Transition1 : RateTransition  Deterministic=off  OutPortSampleTime=Ts1
  Rate Transition11 : RateTransition  Deterministic=off  OutPortSampleTime=Ts1
  Rate Transition2 : RateTransition  Deterministic=off  OutPortSampleTime=Ts1
  single2double2 : DataTypeConversion  OutDataTypeStr=double
  single2double3 : DataTypeConversion  OutDataTypeStr=double
  single2double4 : DataTypeConversion  OutDataTypeStr=double
  u15 : Constant  Value=KI  SampleTime=Ts1
  u16 : Constant  Value=KP  SampleTime=Ts1
  d1 : Outport
  dPI : Outport  Port=2
  wires:
  u16/1 -> PI boost converter controller/4(KP)
  u15/1 -> PI boost converter controller/3(KI)
  Io,opt/1 -> Rate Transition11/1
  Io/1 -> Rate Transition1/1
  Rate Transition11/1 -> single2double3/1
  single2double2/1 -> d1/1
  single2double3/1 -> PI boost converter controller/1(io_ref)
  Rate Transition1/1 -> single2double4/1
  PI boost converter controller/1(dk) -> Rate Transition2/1, dPI/1
  Rate Transition2/1 -> single2double2/1
  single2double4/1 -> PI boost converter controller/2(vo)

== system S_GITHUB/MPPT Algoritm/Start PI boost converter controller ==
  In : Inport
  Compare : simulink/Logic and Bit Operations/Compare To Constant  relop=>=  const=400  OutDataTypeStr=boolean
  D Latch : simulink_extras/Flip Flops/D Latch
      settings: SourceProductName=Simulink  SourceProductBaseCode=SL
  Out : Outport
  wires:
  Compare/1 -> D Latch/2, D Latch/1
  D Latch/1 -> Out/1
  In/1 -> Compare/1

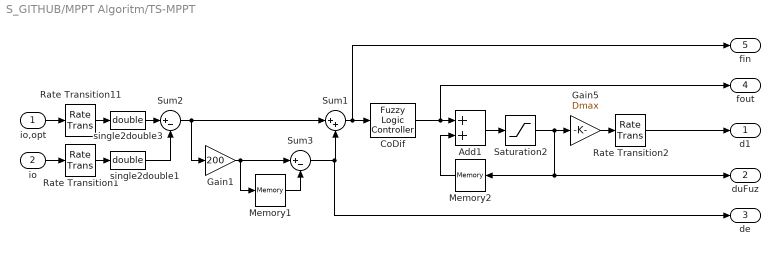
== system S_GITHUB/MPPT Algoritm/TS-MPPT ==
  io,opt : Inport
  io : Inport  Port=2
  Add1 : Sum
  CoDif : fuzblock/Fuzzy Logic  Controller  fis=['TS_MPPT.fis']
  Gain1 : Gain  Gain=200
  Gain5 : Gain  Gain=Dmax
  Memory1 : Memory  InheritSampleTime=on
  Memory2 : Memory  InheritSampleTime=on
  Rate Transition1 : RateTransition  Deterministic=off  OutPortSampleTime=Ts1
  Rate Transition11 : RateTransition  Deterministic=off  OutPortSampleTime=Ts1
  Rate Transition2 : RateTransition  Deterministic=off  OutPortSampleTime=Ts1
  Saturation2 : Saturate  UpperLimit=0.98*Dmax  LowerLimit=0.01*Dmax
  Sum1 : Sum  Inputs=|++
  Sum2 : Sum  Inputs=|+-
  Sum3 : Sum  Inputs=|+-
  single2double1 : DataTypeConversion  OutDataTypeStr=double
  single2double3 : DataTypeConversion  OutDataTypeStr=double
  d1 : Outport
  duFuz : Outport  Port=2
  de : Outport  Port=3
  fout : Outport  Port=4
  fin : Outport  Port=5
  wires:
  Rate Transition2/1 -> d1/1
  Rate Transition11/1 -> single2double3/1
  Gain1/1 -> Memory1/1, Sum3/1
  Memory2/1 -> Add1/2
  single2double3/1 -> Sum2/1
  CoDif/1 -> fout/1, Add1/1
  single2double1/1 -> Sum2/2
  Memory1/1 -> Sum3/2
  Rate Transition1/1 -> single2double1/1
  io,opt/1 -> Rate Transition11/1
  io/1 -> Rate Transition1/1
  Gain5/1 -> Rate Transition2/1
  Add1/1 -> Saturation2/1
  Saturation2/1 -> Gain5/1, duFuz/1, Memory2/1
  Sum2/1 -> Sum1/1, Gain1/1
  Sum3/1 -> Sum1/2, de/1
  Sum1/1 -> fin/1, CoDif/1

== system S_GITHUB/Symmetrical PWM3/Modulation Carrier ==
  Clock : Clock
  Fcn : Fcn  Expr=u*fc-offset
  Lookup Table : Lookup  InputValues=[0 .5 1]  Table=[range(1) range(2) range(1)]  LookUpMeth=Interpolation-Use End Values
  Rounding Function : Rounding
  Subtract : Sum  Inputs=+-
  Unit Delay : UnitDelay  SampleTime=si
  Out : Outport
  wires:
  Lookup Table/1 -> Out/1
  Subtract/1 -> Lookup Table/1
  Rounding Function/1 -> Subtract/2
  Fcn/1 -> Rounding Function/1, Subtract/1
  Clock/1 -> Fcn/1
  Unit Delay/1 -> Unit Delay/1

== system S_GITHUB/Wind turbine (WT)/WT dynamic model ==
  Tm : Inport
  Tg : Inport  Port=2
  Sum : Sum  Inputs=|++
  Transfer function : TransferFcn  Denominator=[(Jm+Jg) Dg]
  Wm : Outport
  wires:
  Tm/1 -> Sum/1
  Tg/1 -> Sum/2
  Sum/1 -> Transfer function/1
  Transfer function/1 -> Wm/1

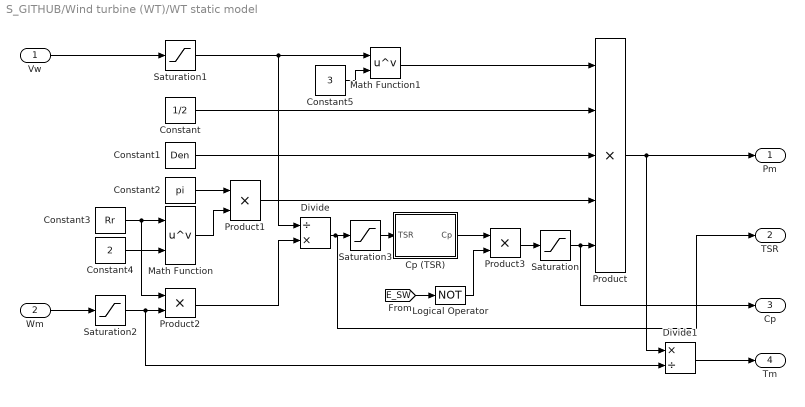
== system S_GITHUB/Wind turbine (WT)/WT static model ==
  Vw : Inport
  Wm : Inport  Port=2
  Constant : Constant  Value=1/2
  Constant1 : Constant  Value=Den
  Constant2 : Constant  Value=pi
  Constant3 : Constant  Value=Rr
  Constant4 : Constant  Value=2
  Constant5 : Constant  Value=3
  Cp (TSR) : MATLAB Function  TreatAsAtomicUnit=on
  Divide : Product  Inputs=/*
  Divide1 : Product  Inputs=*/
  Logical Operator : Logic  Operator=NOT  AllPortsSameDT=off  OutDataTypeStr=boolean
  Math Function : Math  Operator=pow  SaturateOnIntegerOverflow=on
  Math Function1 : Math  Operator=pow  SaturateOnIntegerOverflow=on
  Product : Product  Inputs=5
  Product1 : Product
  Product2 : Product
  Product3 : Product
  Saturation : Saturate  UpperLimit=0.36  LowerLimit=0
  Saturation1 : Saturate  UpperLimit=inf  LowerLimit=0.001
  Saturation2 : Saturate  UpperLimit=inf  LowerLimit=0.001
  Saturation3 : Saturate  UpperLimit=11.68  LowerLimit=0
  Pm : Outport
  TSR : Outport  Port=2
  Cp : Outport  Port=3
  Tm : Outport  Port=4
  wires:
  Math Function1/1 -> Product/1
  Product/1 -> Divide1/1, Pm/1
  Constant5/1 -> Math Function1/2
  Divide1/1 -> Tm/1
  Constant2/1 -> Product1/1
  Product2/1 -> Divide/2
  Constant4/1 -> Math Function/2
  Constant3/1 -> Product2/1, Math Function/1
  Wm/1 -> Saturation2/1
  Math Function/1 -> Product1/2
  Product1/1 -> Product/4
  Constant/1 -> Product/2
  Constant1/1 -> Product/3
  Saturation/1 -> Cp/1, Product/5
  Saturation1/1 -> Divide/1, Math Function1/1
  Saturation2/1 -> Divide1/2, Product2/2
  Divide/1 -> TSR/1, Saturation3/1
  Saturation3/1 -> Cp (TSR)/1(TSR)
  Vw/1 -> Saturation1/1
  Cp (TSR)/1(Cp) -> Product3/1
  Product3/1 -> Saturation/1
  Logical Operator/1 -> Product3/2
  [E_SW] -> Logical Operator/1

== matlab function S_GITHUB/MPPT Algoritm/MPPT algoritm based TSR approach /Io,opt estimator  ==
  data: y input; x output; E output
function [x,E]  = fcn(y)
 
%% Sin consideracion de potencia constante
%3 m/s ---- 16 m/s
% Io_interpolacion=[1 2 3.17 4.74 6.6 8.75 11.6 14.6 18.3 22.5 27.2 32.4 39 47.5];
% Wm_interpolacion=[6.24 8.32 10.4 12.5 14.6 16.6 18.7 20.8 22.9 24.9 27 29.1 31.2 33.3];
%% Consideracion de potencia constante Vw > 14 m/s
%3 m/s ---- 17 m/s
Io_interpolacion=[1 2 3.17 4.74 6.6 8.75 11.6 14.6 18.3 22.5 27.2 32.4 44 54.5 62.3];
Wm_interpolacion=[6.23 8.32 10.4 12.5 14.6 16.6 18.7 20.8 22.9 24.9 27 29.1 31.2 33.3 35.4];
Ir_opt_aux=interp1(Wm_interpolacion,Io_interpolacion,y,'linear');
if(y>35.4)
x=0;
E=1;
elseif(y<6.23)
x=0;
E=1;
else
x=Ir_opt_aux;
E=0;
end

== matlab function S_GITHUB/MPPT Algoritm/MPPT algoritm based TSR approach /Wm,opt computation ==
  data: x input; y output
function y = fcn(x)
Rr      = 2.9343; %Radio [m]
TSR_opt = 6.0997; %Valor óptimo de la velocidad especifica

y = (TSR_opt*x)/Rr;
end

== matlab function S_GITHUB/Wind turbine (WT)/WT static model/Cp (TSR) ==
  data: TSR input; Cp output
function Cp = fcn(TSR)
c1 =   5.953e-07;
c2 =   -2.87e-05;
c3 =   0.0005158;
c4 =   -0.004115;
c5 =     0.01173;
c6 =    0.005831;
c7 =     0.01584;
c8 =    0.004888;
Cp = c1*TSR^7 + c2*TSR^6 + c3*TSR^5 + c4*TSR^4 + c5*TSR^3 + c6*TSR^2 + c7*TSR + c8;

== matlab function S_GITHUB/Wind turbine (WT)/Theoretical maximum power ==
  data: Vw input; Pw output
function Pw = fcn(Vw)
Pw = 1/2*1.225*2.9343^2*3.1416*Vw^3;

== matlab function S_GITHUB/Electrical measurements/Pm,opt ==
  data: Vw input; Pw output
function Pw = fcn(Vw)
Pw = 1/2*1.225*2.9343^2*3.1416*Vw^3*0.349;

== matlab function S_GITHUB/MPPT Algoritm/PI-MPPT/PI boost converter controller ==
  data: io_ref input; dk output; vo input; KI input; KP input
function dk = fcn(io_ref, vo, KI, KP)

 %Valores iniciales de las conStantes del controlador
 persistent  ek uk
 persistent  ek_1 uk_1
 if isempty(ek)
    ek =0;
    uk =0;
    ek_1 =0;
    uk_1 =0;
 end
ek=io_ref-vo;
uk=ek*(KP+KI)-ek_1*KP+uk_1;
%uk=KP*ek+KI*ek+KI*ek_1;
if(uk>(0.95))
    uk=0.95;
end
if(uk<0.01)
    uk=0.01;
end
ek_1=ek;
uk_1=uk;
dk=uk;
end
